simulink model "simulationComplete"  (R2024a)
settings: Solver=FixedStepAuto  StartTime=0.0  StopTime=1500  FixedStep=1E-4  RelTol=1e-3
values from neighbouring files (symbols this model uses):
  gamma_p = 0.1    [simulationParameters.m]    (also in untitled10.m)
  Kp_init = 1    [simulationParameters.m]    (also in untitled10.m)
  x = yout{5}.Values    [plottts.m]
undefined symbols (not defined in the file or in its folder): esti, init, motor, sat
settings Model: Creator=b_ant  LastModifiedBy=workstation

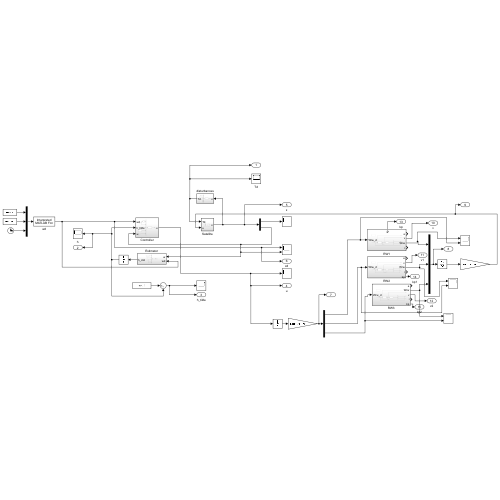
[thumbnail: Simulink's stored preview of the top-level diagram]
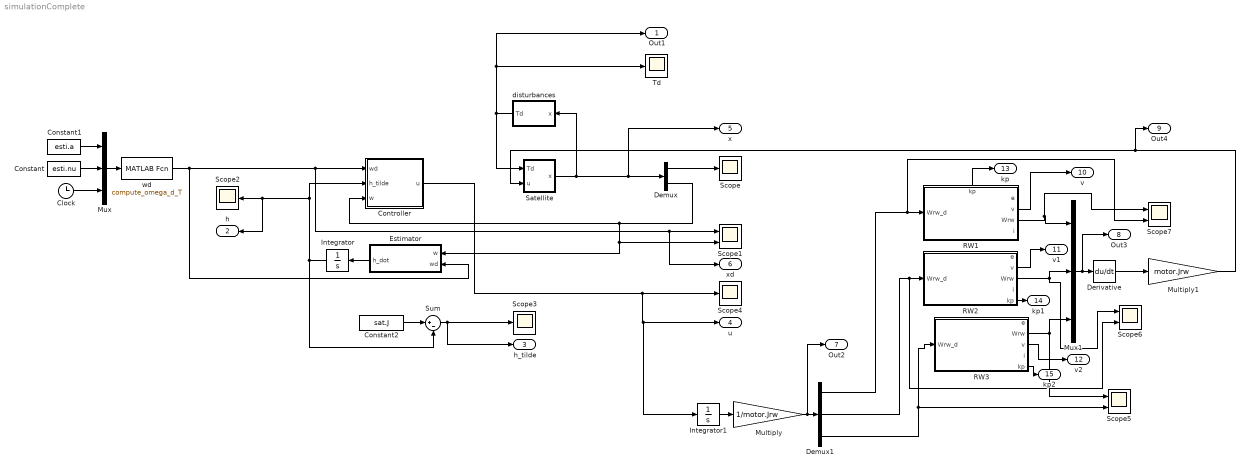
== system simulationComplete ==
  Clock : Clock
  Constant : Constant  Value=esti.nu
  Constant1 : Constant  Value=esti.a
  Constant2 : Constant  Value=sat.J
  Controller : Subsystem
  Demux : Demux  Outputs=2
  Demux1 : Demux  Outputs=3
  Derivative : Derivative
  Estimator : Subsystem
  Integrator : Integrator
  Integrator1 : Integrator
  Multiply : Gain  Gain=1/motor.Jrw
  Multiply1 : Gain  Gain=motor.Jrw
  Mux : Mux  Inputs=3
  Mux1 : Mux  Inputs=3
  RW1 : Subsystem
      settings: PortSchema="{\"entries\":[{\"content\":{\"sides\":[{\"content\":{\"connectorIds\":[\"In1\"]},\"type\":\"ConnectorPlacement.EquallySpacedRectSide\",\"uuid\":\"676f5149-fe3d-4701-b2d2-e4428c1af590\"},{\"content\":{\"connectorIds\":[\"Out1\",\"Out2\",\"Out3\",\"Out4\"],\"side\":\"RIGHT\"},\"type\":\"ConnectorPlacement.EquallySpacedRectSide\",\"uuid\":\"0b9cb26b-9812-4b00-bfdf-ae8b5656d0ce\"},{\"content\":{\"connectorIds\":[\"Out5\"],\"side\":\"TOP\"},\"type\":\"ConnectorPlacement.EquallySpacedRectSide\",\"uuid\":\"75ccec44-caa4-4b18-8247-0b69eee9b1da\"}]},\"type\":\"ConnectorPlacement.EquallySpacedConnector\",\"uuid\":\"c8c35d5e-ed2c-47c8-89dc-6ef741e7efc5\"}],\"packageUris\":[\"http://schema.mathworks.com/mf0/Connector/R2020b\"],\"version\":\"1.0\"}"
  RW2 : Subsystem
  RW3 : Subsystem
  Satellite : Subsystem
  Scope{,2..4} (4 alike) : Scope
  Scope{1,5..7} (4 alike) : Scope  NumInputPorts=2
  Sum : Sum  Inputs=|+-
  Td : Scope
  disturbances : Subsystem
  wd : MATLABFcn  MATLABFcn=compute_omega_d_T
  Out1 : Outport
  h : Outport  Port=2
  h_tilde : Outport  Port=3
  u : Outport  Port=4
  x : Outport  Port=5
  xd : Outport  Port=6
  Out2 : Outport  Port=7
  Out3 : Outport  Port=8
  Out4 : Outport  Port=9
  v : Outport  Port=10
  v1 : Outport  Port=11
  v2 : Outport  Port=12
  kp : Outport  Port=13
  kp1 : Outport  Port=14
  kp2 : Outport  Port=15
  wires:
  Controller/1(u) -> Integrator1/1, u/1, Scope4/1
  Sum/1 -> h_tilde/1, Scope3/1
  Clock/1 -> Mux/3
  Constant2/1 -> Sum/1
  Constant/1 -> Mux/2
  Mux/1 -> wd/1
  Constant1/1 -> Mux/1
  Integrator/1 -> Controller/2(h_tilde), h/1, Scope2/1, Sum/2
  Estimator/1(h_dot) -> Integrator/1
  Satellite/1(x) -> x/1, Demux/1, disturbances/1(x)
  Demux/1 -> Scope/1
  Demux/2 -> Estimator/1(w), Scope1/2, Controller/3(w)
  disturbances/1(Td) -> Out1/1, Td/1, Satellite/1(Td)
  wd/1 -> xd/1, Scope1/1, Controller/1(wd), Estimator/2(wd)
  Integrator1/1 -> Multiply/1
  Multiply/1 -> Out2/1, Demux1/1
  Demux1/1 -> Scope7/2, RW1/1(Wrw_d)
  Demux1/2 -> Scope6/2, RW2/1(Wrw_d)
  Demux1/3 -> Scope5/2, RW3/1(Wrw_d)
  RW1/3(Wrw) -> Scope7/1, Mux1/1
  RW2/3(Wrw) -> Scope6/1, Mux1/2
  Mux1/1 -> Out3/1, Derivative/1
  Derivative/1 -> Multiply1/1
  Multiply1/1 -> Out4/1, Satellite/2(u)
  RW3/2(Wrw) -> Scope5/1, Mux1/3
  RW1/2(v) -> v/1
  RW2/2(v) -> v1/1
  RW3/3(v) -> v2/1
  RW1/5(kp) -> kp/1
  RW2/5(kp) -> kp1/1
  RW3/5(kp) -> kp2/1

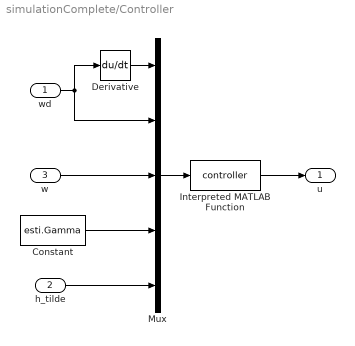
== system simulationComplete/Controller ==
  wd : Inport
  h_tilde : Inport  Port=2
  w : Inport  Port=3
  Constant : Constant  Value=esti.Gamma
  Derivative : Derivative
  Interpreted MATLAB Function : MATLABFcn  MATLABFcn=controller
  Mux : Mux  Inputs=5
  u : Outport
  wires:
  h_tilde/1 -> Mux/5
  w/1 -> Mux/3
  Constant/1 -> Mux/4
  Interpreted MATLAB Function/1 -> u/1
  Mux/1 -> Interpreted MATLAB Function/1
  wd/1 -> Mux/2, Derivative/1
  Derivative/1 -> Mux/1

== system simulationComplete/Estimator ==
  w : Inport
  wd : Inport  Port=2
  Constant : Constant  Value=esti.gamma  VectorParams1D=off
  Derivative : Derivative
  Interpreted MATLAB Function : MATLABFcn  MATLABFcn=estimator
  Mux : Mux
  h_dot : Outport
  wires:
  Mux/1 -> Interpreted MATLAB Function/1
  Derivative/1 -> Mux/4
  wd/1 -> Derivative/1, Mux/3
  w/1 -> Mux/2
  Interpreted MATLAB Function/1 -> h_dot/1
  Constant/1 -> Mux/1

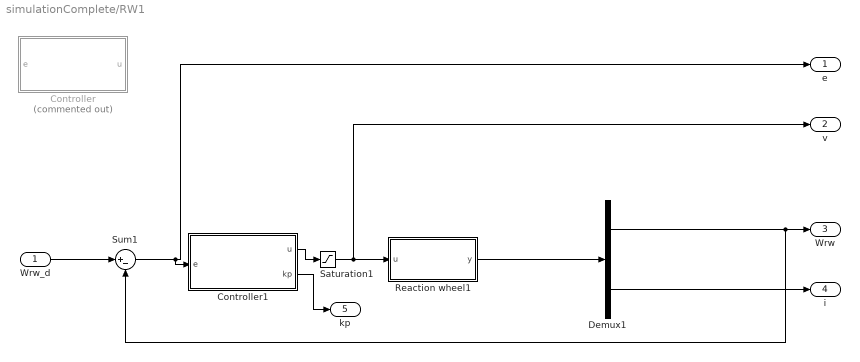
== system simulationComplete/RW1 ==
  Wrw_d : Inport
  Controller : Subsystem  Commented=on
  Controller1 : Subsystem
  Demux1 : Demux  Outputs=2
  Reaction wheel1 : Subsystem
  Saturation1 : Saturate  UpperLimit=Inf  LowerLimit=-Inf
  Sum1 : Sum  Inputs=|+-
  e : Outport
  v : Outport  Port=2
  Wrw : Outport  Port=3
  i : Outport  Port=4
  kp : Outport  Port=5
  wires:
  Demux1/1 -> Sum1/2, Wrw/1
  Demux1/2 -> i/1
  Reaction wheel1/1(y) -> Demux1/1
  Sum1/1 -> e/1, Controller1/1(e)
  Saturation1/1 -> v/1, Reaction wheel1/1(u)
  Wrw_d/1 -> Sum1/1
  Controller1/1(u) -> Saturation1/1
  Controller1/2(kp) -> kp/1

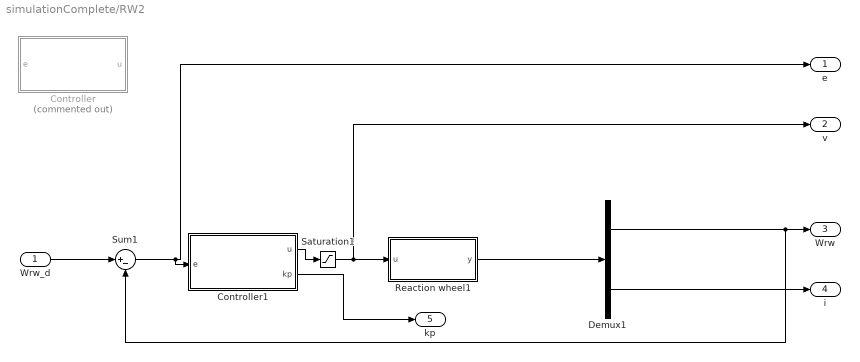
== system simulationComplete/RW2 ==
  Wrw_d : Inport
  Controller : Subsystem  Commented=on
  Controller1 : Subsystem
  Demux1 : Demux  Outputs=2
  Reaction wheel1 : Subsystem
  Saturation1 : Saturate  UpperLimit=Inf  LowerLimit=-Inf
  Sum1 : Sum  Inputs=|+-
  e : Outport
  v : Outport  Port=2
  Wrw : Outport  Port=3
  i : Outport  Port=4
  kp : Outport  Port=5
  wires:
  Demux1/1 -> Sum1/2, Wrw/1
  Demux1/2 -> i/1
  Reaction wheel1/1(y) -> Demux1/1
  Sum1/1 -> e/1, Controller1/1(e)
  Saturation1/1 -> v/1, Reaction wheel1/1(u)
  Wrw_d/1 -> Sum1/1
  Controller1/1(u) -> Saturation1/1
  Controller1/2(kp) -> kp/1

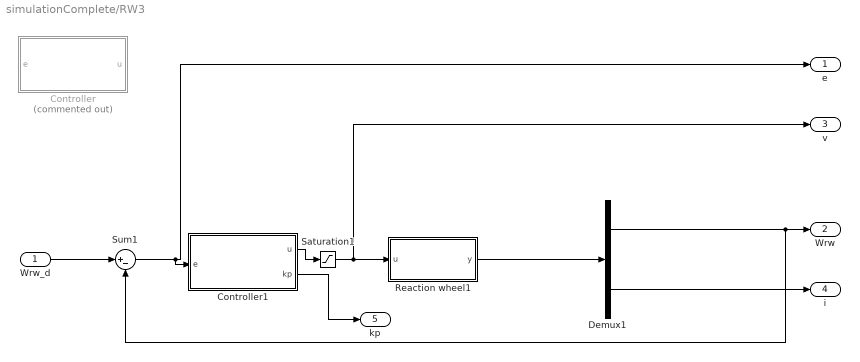
== system simulationComplete/RW3 ==
  Wrw_d : Inport
  Controller : Subsystem  Commented=on
  Controller1 : Subsystem
  Demux1 : Demux  Outputs=2
  Reaction wheel1 : Subsystem
  Saturation1 : Saturate  UpperLimit=Inf  LowerLimit=-Inf
  Sum1 : Sum  Inputs=|+-
  e : Outport
  Wrw : Outport  Port=2
  v : Outport  Port=3
  i : Outport  Port=4
  kp : Outport  Port=5
  wires:
  Demux1/1 -> Sum1/2, Wrw/1
  Demux1/2 -> i/1
  Reaction wheel1/1(y) -> Demux1/1
  Sum1/1 -> e/1, Controller1/1(e)
  Saturation1/1 -> v/1, Reaction wheel1/1(u)
  Wrw_d/1 -> Sum1/1
  Controller1/1(u) -> Saturation1/1
  Controller1/2(kp) -> kp/1

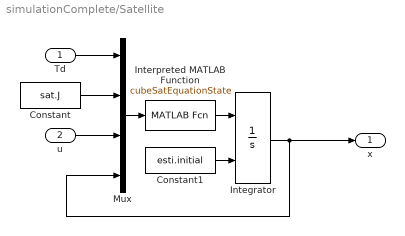
== system simulationComplete/Satellite ==
  Td : Inport
  u : Inport  Port=2
  Constant : Constant  Value=sat.J
  Constant1 : Constant  Value=esti.initial
  Integrator : Integrator  InitialConditionSource=external
  Interpreted MATLAB Function : MATLABFcn  MATLABFcn=cubeSatEquationState
  Mux : Mux
  x : Outport
  wires:
  u/1 -> Mux/3
  Integrator/1 -> x/1, Mux/4
  Mux/1 -> Interpreted MATLAB Function/1
  Interpreted MATLAB Function/1 -> Integrator/1
  Constant/1 -> Mux/2
  Td/1 -> Mux/1
  Constant1/1 -> Integrator/2

== system simulationComplete/disturbances ==
  x : Inport
  Constant1 : Constant  Value=sat.m_sat
  Constant3 : Constant  Value=sat.cg
  Constant4 : Constant  Value=sat.alpha
  Constant5 : Constant  Value=sat.miss
  Interpreted MATLAB Function : MATLABFcn  MATLABFcn=disturbances
  Mux1 : Mux  Inputs=5
  Td : Outport
  wires:
  Constant5/1 -> Mux1/4
  Constant3/1 -> Mux1/2
  Constant4/1 -> Mux1/3
  Mux1/1 -> Interpreted MATLAB Function/1
  Interpreted MATLAB Function/1 -> Td/1
  x/1 -> Mux1/1
  Constant1/1 -> Mux1/5

== system simulationComplete/RW1/Controller ==
  e : Inport
  Adaptation Law : Subsystem  mask{alpha=x.alpha, beta=x.beta, epsilon=x.epsilon, n=x.n, kd0=x.kd_init, ki0=x.ki_init, kp0=x.kp_init}
      mask prompts: kd0 "kd_0:"; ki0 "ki_0:"; kp0 "kp_0:"
      mask TypeOptions alpha: alpha/Value
      mask TypeOptions beta: beta/Value
      mask TypeOptions epsilon: epsilon/Value
      mask TypeOptions n: n/Value
      mask TypeOptions kd0: kd0/Value
      mask TypeOptions ki0: ki0/Value
      mask TypeOptions kp0: kp0/Value
  Display : Display
  PID controller : Subsystem
  Scope : Scope
  Sliding surface : Subsystem  mask{Gain=x.lambda}
      mask prompts: Gain "Simulink:blkprm_prompts:GainGain"
      mask TypeOptions Gain: Gain/Gain
      mask DialogControl Gain Prompt: Gain:
  error subsystem : Subsystem
  u : Outport
  wires:
  Sliding surface/1(s) -> Adaptation Law/2(s)
  Sliding surface/2(s_dot) -> Adaptation Law/3(s_dot)
  PID controller/1(u) -> u/1
  Adaptation Law/1(theta) -> Scope/1, Display/1, PID controller/1(theta)
  error subsystem/1(MyPi) -> PID controller/2(MyPi), Adaptation Law/1(myPi)
  e/1 -> error subsystem/1(e), Sliding surface/1(e)

== system simulationComplete/RW1/Controller1 ==
  e : Inport
  Constant : Constant  Value=gamma_p
  Integrator : Integrator  InitialCondition=Kp_init
  MATLAB Function : MATLAB Function  TreatAsAtomicUnit=on
  MATLAB Function1 : MATLAB Function  TreatAsAtomicUnit=on
  u : Outport
  kp : Outport  Port=2
  wires:
  MATLAB Function/1(u) -> u/1
  MATLAB Function1/1(kp_dot) -> Integrator/1
  Integrator/1 -> kp/1, MATLAB Function/1(Kp)
  e/1 -> MATLAB Function/2(error), MATLAB Function1/2(error)
  Constant/1 -> MATLAB Function1/1(gamma_p)

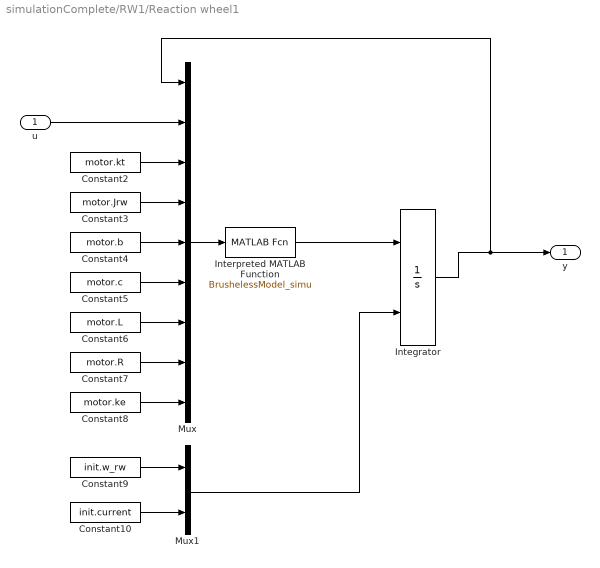
== system simulationComplete/RW1/Reaction wheel1 ==
  u : Inport
  Constant10 : Constant  Value=init.current
  Constant2 : Constant  Value=motor.kt
  Constant3 : Constant  Value=motor.Jrw
  Constant4 : Constant  Value=motor.b
  Constant5 : Constant  Value=motor.c
  Constant6 : Constant  Value=motor.L
  Constant7 : Constant  Value=motor.R
  Constant8 : Constant  Value=motor.ke
  Constant9 : Constant  Value=init.w_rw
  Integrator : Integrator  InitialConditionSource=external
  Interpreted MATLAB Function : MATLABFcn  MATLABFcn=BrushelessModel_simu  OutputDimensions=2
  Mux : Mux  Inputs=9
  Mux1 : Mux  Inputs=2
  y : Outport
  wires:
  Interpreted MATLAB Function/1 -> Integrator/1
  Constant8/1 -> Mux/9
  Integrator/1 -> Mux/1, y/1
  Constant10/1 -> Mux1/2
  Constant9/1 -> Mux1/1
  Mux/1 -> Interpreted MATLAB Function/1
  Mux1/1 -> Integrator/2
  u/1 -> Mux/2
  Constant2/1 -> Mux/3
  Constant3/1 -> Mux/4
  Constant4/1 -> Mux/5
  Constant5/1 -> Mux/6
  Constant6/1 -> Mux/7
  Constant7/1 -> Mux/8

== system simulationComplete/RW2/Controller ==
  e : Inport
  Adaptation Law : Subsystem  mask{alpha=x.alpha, beta=x.beta, epsilon=x.epsilon, n=x.n, kd0=x.kd_init, ki0=x.ki_init, kp0=x.kp_init}
      mask prompts: kd0 "kd_0:"; ki0 "ki_0:"; kp0 "kp_0:"
      mask TypeOptions alpha: alpha/Value
      mask TypeOptions beta: beta/Value
      mask TypeOptions epsilon: epsilon/Value
      mask TypeOptions n: n/Value
      mask TypeOptions kd0: kd0/Value
      mask TypeOptions ki0: ki0/Value
      mask TypeOptions kp0: kp0/Value
  Display : Display
  PID controller : Subsystem
  Scope : Scope
  Sliding surface : Subsystem  mask{Gain=x.lambda}
      mask prompts: Gain "Simulink:blkprm_prompts:GainGain"
      mask TypeOptions Gain: Gain/Gain
      mask DialogControl Gain Prompt: Gain:
  error subsystem : Subsystem
  u : Outport
  wires:
  Sliding surface/1(s) -> Adaptation Law/2(s)
  Sliding surface/2(s_dot) -> Adaptation Law/3(s_dot)
  PID controller/1(u) -> u/1
  Adaptation Law/1(theta) -> Scope/1, Display/1, PID controller/1(theta)
  error subsystem/1(MyPi) -> PID controller/2(MyPi), Adaptation Law/1(myPi)
  e/1 -> error subsystem/1(e), Sliding surface/1(e)

== system simulationComplete/RW2/Controller1 ==
  e : Inport
  Constant : Constant  Value=gamma_p
  Integrator : Integrator  InitialCondition=Kp_init
  MATLAB Function : MATLAB Function  TreatAsAtomicUnit=on
  MATLAB Function1 : MATLAB Function  TreatAsAtomicUnit=on
  u : Outport
  kp : Outport  Port=2
  wires:
  MATLAB Function/1(u) -> u/1
  MATLAB Function1/1(kp_dot) -> Integrator/1
  Integrator/1 -> kp/1, MATLAB Function/1(Kp)
  e/1 -> MATLAB Function/2(error), MATLAB Function1/2(error)
  Constant/1 -> MATLAB Function1/1(gamma_p)

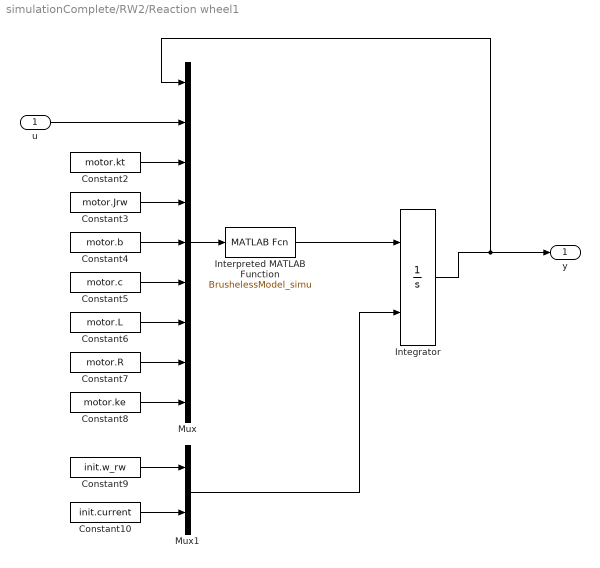
== system simulationComplete/RW2/Reaction wheel1 ==
  u : Inport
  Constant10 : Constant  Value=init.current
  Constant2 : Constant  Value=motor.kt
  Constant3 : Constant  Value=motor.Jrw
  Constant4 : Constant  Value=motor.b
  Constant5 : Constant  Value=motor.c
  Constant6 : Constant  Value=motor.L
  Constant7 : Constant  Value=motor.R
  Constant8 : Constant  Value=motor.ke
  Constant9 : Constant  Value=init.w_rw
  Integrator : Integrator  InitialConditionSource=external
  Interpreted MATLAB Function : MATLABFcn  MATLABFcn=BrushelessModel_simu  OutputDimensions=2
  Mux : Mux  Inputs=9
  Mux1 : Mux  Inputs=2
  y : Outport
  wires:
  Interpreted MATLAB Function/1 -> Integrator/1
  Constant8/1 -> Mux/9
  Integrator/1 -> Mux/1, y/1
  Constant10/1 -> Mux1/2
  Constant9/1 -> Mux1/1
  Mux/1 -> Interpreted MATLAB Function/1
  Mux1/1 -> Integrator/2
  u/1 -> Mux/2
  Constant2/1 -> Mux/3
  Constant3/1 -> Mux/4
  Constant4/1 -> Mux/5
  Constant5/1 -> Mux/6
  Constant6/1 -> Mux/7
  Constant7/1 -> Mux/8

== system simulationComplete/RW3/Controller ==
  e : Inport
  Adaptation Law : Subsystem  mask{alpha=x.alpha, beta=x.beta, epsilon=x.epsilon, n=x.n, kd0=x.kd_init, ki0=x.ki_init, kp0=x.kp_init}
      mask prompts: kd0 "kd_0:"; ki0 "ki_0:"; kp0 "kp_0:"
      mask TypeOptions alpha: alpha/Value
      mask TypeOptions beta: beta/Value
      mask TypeOptions epsilon: epsilon/Value
      mask TypeOptions n: n/Value
      mask TypeOptions kd0: kd0/Value
      mask TypeOptions ki0: ki0/Value
      mask TypeOptions kp0: kp0/Value
  Display : Display
  PID controller : Subsystem
  Scope : Scope
  Sliding surface : Subsystem  mask{Gain=x.lambda}
      mask prompts: Gain "Simulink:blkprm_prompts:GainGain"
      mask TypeOptions Gain: Gain/Gain
      mask DialogControl Gain Prompt: Gain:
  error subsystem : Subsystem
  u : Outport
  wires:
  Sliding surface/1(s) -> Adaptation Law/2(s)
  Sliding surface/2(s_dot) -> Adaptation Law/3(s_dot)
  PID controller/1(u) -> u/1
  Adaptation Law/1(theta) -> Scope/1, Display/1, PID controller/1(theta)
  error subsystem/1(MyPi) -> PID controller/2(MyPi), Adaptation Law/1(myPi)
  e/1 -> error subsystem/1(e), Sliding surface/1(e)

== system simulationComplete/RW3/Controller1 ==
  e : Inport
  Constant : Constant  Value=gamma_p
  Integrator : Integrator  InitialCondition=Kp_init
  MATLAB Function : MATLAB Function  TreatAsAtomicUnit=on
  MATLAB Function1 : MATLAB Function  TreatAsAtomicUnit=on
  u : Outport
  kp : Outport  Port=2
  wires:
  MATLAB Function/1(u) -> u/1
  MATLAB Function1/1(kp_dot) -> Integrator/1
  Integrator/1 -> kp/1, MATLAB Function/1(Kp)
  e/1 -> MATLAB Function/2(error), MATLAB Function1/2(error)
  Constant/1 -> MATLAB Function1/1(gamma_p)

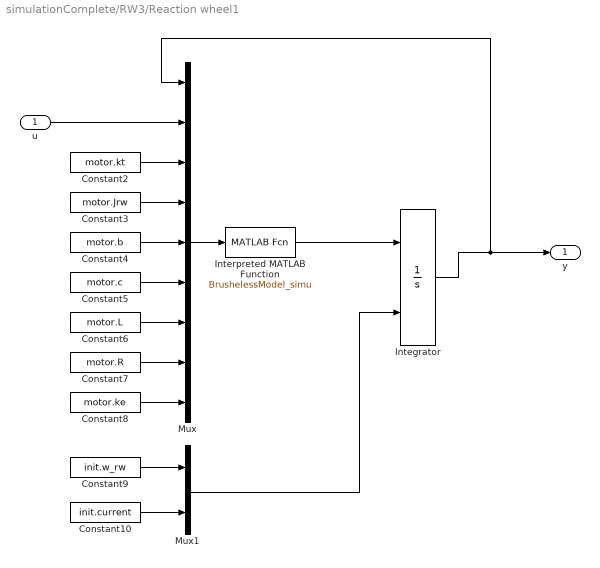
== system simulationComplete/RW3/Reaction wheel1 ==
  u : Inport
  Constant10 : Constant  Value=init.current
  Constant2 : Constant  Value=motor.kt
  Constant3 : Constant  Value=motor.Jrw
  Constant4 : Constant  Value=motor.b
  Constant5 : Constant  Value=motor.c
  Constant6 : Constant  Value=motor.L
  Constant7 : Constant  Value=motor.R
  Constant8 : Constant  Value=motor.ke
  Constant9 : Constant  Value=init.w_rw
  Integrator : Integrator  InitialConditionSource=external
  Interpreted MATLAB Function : MATLABFcn  MATLABFcn=BrushelessModel_simu  OutputDimensions=2
  Mux : Mux  Inputs=9
  Mux1 : Mux  Inputs=2
  y : Outport
  wires:
  Interpreted MATLAB Function/1 -> Integrator/1
  Constant8/1 -> Mux/9
  Integrator/1 -> Mux/1, y/1
  Constant10/1 -> Mux1/2
  Constant9/1 -> Mux1/1
  Mux/1 -> Interpreted MATLAB Function/1
  Mux1/1 -> Integrator/2
  u/1 -> Mux/2
  Constant2/1 -> Mux/3
  Constant3/1 -> Mux/4
  Constant4/1 -> Mux/5
  Constant5/1 -> Mux/6
  Constant6/1 -> Mux/7
  Constant7/1 -> Mux/8

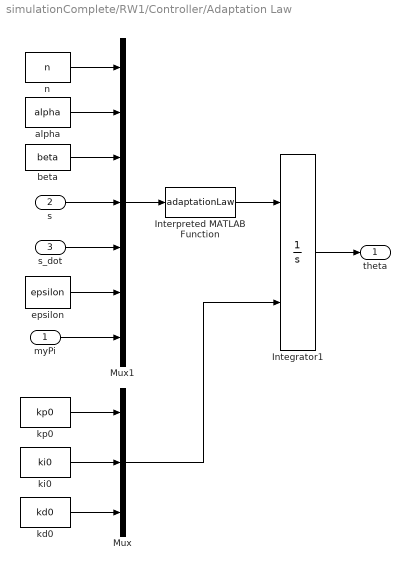
== system simulationComplete/RW1/Controller/Adaptation Law ==
  myPi : Inport
  s : Inport  Port=2
  s_dot : Inport  Port=3
  Integrator1 : Integrator  InitialConditionSource=external  InitialCondition=[1.460477259865257e-04,6.548069875818259e-05,0]
  Interpreted MATLAB Function : MATLABFcn  MATLABFcn=adaptationLaw
  Mux : Mux  Inputs=3
  Mux1 : Mux  Inputs=7
  alpha : Constant  Value=alpha
  beta : Constant  Value=beta
  epsilon : Constant  Value=epsilon
  kd0 : Constant  Value=kd0
  ki0 : Constant  Value=ki0
  kp0 : Constant  Value=kp0
  n : Constant  Value=n
  theta : Outport
  wires:
  alpha/1 -> Mux1/2
  Interpreted MATLAB Function/1 -> Integrator1/1
  myPi/1 -> Mux1/7
  s/1 -> Mux1/4
  epsilon/1 -> Mux1/6
  Integrator1/1 -> theta/1
  s_dot/1 -> Mux1/5
  beta/1 -> Mux1/3
  Mux1/1 -> Interpreted MATLAB Function/1
  n/1 -> Mux1/1
  ki0/1 -> Mux/2
  Mux/1 -> Integrator1/2
  kp0/1 -> Mux/1
  kd0/1 -> Mux/3

== system simulationComplete/RW1/Controller/PID controller ==
  theta : Inport
  MyPi : Inport  Port=2
  Interpreted MATLAB Function1 : MATLABFcn  MATLABFcn=controlLaw  OutputDimensions=1
  Mux2 : Mux  Inputs=2
  u : Outport
  wires:
  Mux2/1 -> Interpreted MATLAB Function1/1
  theta/1 -> Mux2/1
  Interpreted MATLAB Function1/1 -> u/1
  MyPi/1 -> Mux2/2

== system simulationComplete/RW1/Controller/Sliding surface ==
  note: s
  note: e
  e : Inport
  Add : Sum
  Derivative : Derivative
  Derivative1 : Derivative
  Gain : Gain  Gain=Gain
  s : Outport
  s_dot : Outport  Port=2
  wires:
  Add/1 -> s/1, Derivative1/1
  Gain/1 -> Add/1
  e/1 -> Derivative/1, Gain/1
  Derivative/1 -> Add/2
  Derivative1/1 -> s_dot/1

== system simulationComplete/RW1/Controller/error subsystem ==
  e : Inport
  Derivative : Derivative
  Integrator : Integrator
  Mux : Mux  Inputs=3
  MyPi : Outport
  wires:
  e/1 -> Derivative/1, Mux/1, Integrator/1
  Integrator/1 -> Mux/2
  Mux/1 -> MyPi/1
  Derivative/1 -> Mux/3

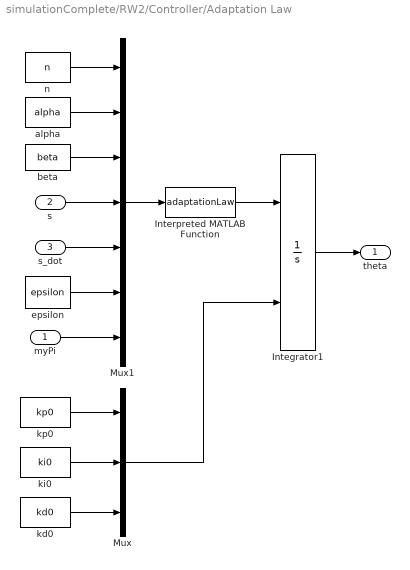
== system simulationComplete/RW2/Controller/Adaptation Law ==
  myPi : Inport
  s : Inport  Port=2
  s_dot : Inport  Port=3
  Integrator1 : Integrator  InitialConditionSource=external  InitialCondition=[1.460477259865257e-04,6.548069875818259e-05,0]
  Interpreted MATLAB Function : MATLABFcn  MATLABFcn=adaptationLaw
  Mux : Mux  Inputs=3
  Mux1 : Mux  Inputs=7
  alpha : Constant  Value=alpha
  beta : Constant  Value=beta
  epsilon : Constant  Value=epsilon
  kd0 : Constant  Value=kd0
  ki0 : Constant  Value=ki0
  kp0 : Constant  Value=kp0
  n : Constant  Value=n
  theta : Outport
  wires:
  alpha/1 -> Mux1/2
  Interpreted MATLAB Function/1 -> Integrator1/1
  myPi/1 -> Mux1/7
  s/1 -> Mux1/4
  epsilon/1 -> Mux1/6
  Integrator1/1 -> theta/1
  s_dot/1 -> Mux1/5
  beta/1 -> Mux1/3
  Mux1/1 -> Interpreted MATLAB Function/1
  n/1 -> Mux1/1
  ki0/1 -> Mux/2
  Mux/1 -> Integrator1/2
  kp0/1 -> Mux/1
  kd0/1 -> Mux/3

== system simulationComplete/RW2/Controller/PID controller ==
  theta : Inport
  MyPi : Inport  Port=2
  Interpreted MATLAB Function1 : MATLABFcn  MATLABFcn=controlLaw  OutputDimensions=1
  Mux2 : Mux  Inputs=2
  u : Outport
  wires:
  Mux2/1 -> Interpreted MATLAB Function1/1
  theta/1 -> Mux2/1
  Interpreted MATLAB Function1/1 -> u/1
  MyPi/1 -> Mux2/2

== system simulationComplete/RW2/Controller/Sliding surface ==
  note: s
  note: e
  e : Inport
  Add : Sum
  Derivative : Derivative
  Derivative1 : Derivative
  Gain : Gain  Gain=Gain
  s : Outport
  s_dot : Outport  Port=2
  wires:
  Add/1 -> s/1, Derivative1/1
  Gain/1 -> Add/1
  e/1 -> Derivative/1, Gain/1
  Derivative/1 -> Add/2
  Derivative1/1 -> s_dot/1

== system simulationComplete/RW2/Controller/error subsystem ==
  e : Inport
  Derivative : Derivative
  Integrator : Integrator
  Mux : Mux  Inputs=3
  MyPi : Outport
  wires:
  e/1 -> Derivative/1, Mux/1, Integrator/1
  Integrator/1 -> Mux/2
  Mux/1 -> MyPi/1
  Derivative/1 -> Mux/3

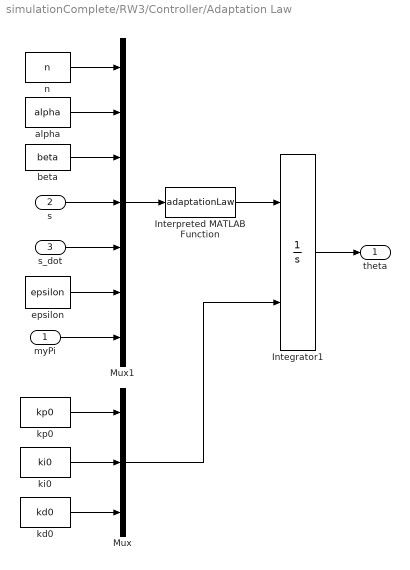
== system simulationComplete/RW3/Controller/Adaptation Law ==
  myPi : Inport
  s : Inport  Port=2
  s_dot : Inport  Port=3
  Integrator1 : Integrator  InitialConditionSource=external  InitialCondition=[1.460477259865257e-04,6.548069875818259e-05,0]
  Interpreted MATLAB Function : MATLABFcn  MATLABFcn=adaptationLaw
  Mux : Mux  Inputs=3
  Mux1 : Mux  Inputs=7
  alpha : Constant  Value=alpha
  beta : Constant  Value=beta
  epsilon : Constant  Value=epsilon
  kd0 : Constant  Value=kd0
  ki0 : Constant  Value=ki0
  kp0 : Constant  Value=kp0
  n : Constant  Value=n
  theta : Outport
  wires:
  alpha/1 -> Mux1/2
  Interpreted MATLAB Function/1 -> Integrator1/1
  myPi/1 -> Mux1/7
  s/1 -> Mux1/4
  epsilon/1 -> Mux1/6
  Integrator1/1 -> theta/1
  s_dot/1 -> Mux1/5
  beta/1 -> Mux1/3
  Mux1/1 -> Interpreted MATLAB Function/1
  n/1 -> Mux1/1
  ki0/1 -> Mux/2
  Mux/1 -> Integrator1/2
  kp0/1 -> Mux/1
  kd0/1 -> Mux/3

== system simulationComplete/RW3/Controller/PID controller ==
  theta : Inport
  MyPi : Inport  Port=2
  Interpreted MATLAB Function1 : MATLABFcn  MATLABFcn=controlLaw  OutputDimensions=1
  Mux2 : Mux  Inputs=2
  u : Outport
  wires:
  Mux2/1 -> Interpreted MATLAB Function1/1
  theta/1 -> Mux2/1
  Interpreted MATLAB Function1/1 -> u/1
  MyPi/1 -> Mux2/2

== system simulationComplete/RW3/Controller/Sliding surface ==
  note: s
  note: e
  e : Inport
  Add : Sum
  Derivative : Derivative
  Derivative1 : Derivative
  Gain : Gain  Gain=Gain
  s : Outport
  s_dot : Outport  Port=2
  wires:
  Add/1 -> s/1, Derivative1/1
  Gain/1 -> Add/1
  e/1 -> Derivative/1, Gain/1
  Derivative/1 -> Add/2
  Derivative1/1 -> s_dot/1

== system simulationComplete/RW3/Controller/error subsystem ==
  e : Inport
  Derivative : Derivative
  Integrator : Integrator
  Mux : Mux  Inputs=3
  MyPi : Outport
  wires:
  e/1 -> Derivative/1, Mux/1, Integrator/1
  Integrator/1 -> Mux/2
  Mux/1 -> MyPi/1
  Derivative/1 -> Mux/3

== matlab function simulationComplete/RW1/Controller1/MATLAB Function ==
  data: Kp input; u output; error input
function u = P_control(Kp,error)
    u = Kp * error;
end

== matlab function simulationComplete/RW2/Controller1/MATLAB Function ==
  data: Kp input; u output; error input
function u = P_control(Kp,error)
    u = Kp * error;
end

== matlab function simulationComplete/RW2/Controller1/MATLAB Function1 ==
  data: gamma_p input; kp_dot output; error input
function kp_dot = fcn(gamma_p,error)
    kp_dot = gamma_p * abs(error);
end

== matlab function simulationComplete/RW3/Controller1/MATLAB Function ==
  data: Kp input; u output; error input
function u = P_control(Kp,error)
    u = Kp * error;
end

== matlab function simulationComplete/RW3/Controller1/MATLAB Function1 ==
  data: gamma_p input; kp_dot output; error input
function kp_dot = fcn(gamma_p,error)
    kp_dot = gamma_p * abs(error);
end

== matlab function simulationComplete/RW1/Controller1/MATLAB Function1 ==
  data: gamma_p input; kp_dot output; error input
function kp_dot = fcn(gamma_p,error)
    kp_dot = gamma_p * abs(error);
end
